simulink model "survillence"  (Simulink 7.9)
settings: Solver=ode45  StartTime=0.0  StopTime=100.0  RelTol=1e-3
undefined symbols (not defined in the file): jet
libraries: visionsinks x2, visionanalysis x1, dspvision x1
settings Model: Creator=user  LastModifiedBy=user

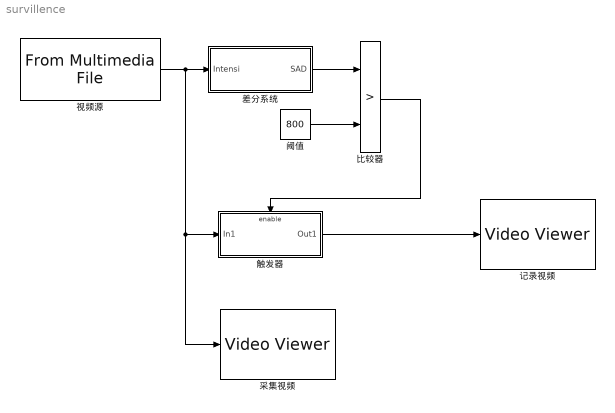
== system survillence ==
  差分系统 : Subsystem
  比较器 : RelationalOperator  Operator=>  OutDataTypeStr=boolean
  视频源 : dspvision/From Multimedia File  inputFilename=vipmen.avi  loop=on  numPlays=inf  outputStreams=Video only  videoDataType=double  audioDataType=int16  inheritSampleTime=on  userDefinedSampleTime=1/30  noAudioOutput=off  isIntensityVideo=off  fourcc=Intensity  colorVideoFormat=One multidimensional signal  outputEOF=off  dataOrg=Column-major  audioFrameSize=1024  computeAudioFrameSize=off  outSamplingMode=Sample based
  触发器 : Subsystem
  记录视频 : visionsinks/Video Viewer  inputType=Obsolete7b  imagePorts=One multidimensional signal  useColorMap=off  colormapValue=jet(256)  specRange=off  minInputVal=0  maxInputVal=255  FigPos=[601 774 410 300]  AxisZoom=on  trueSizedOnce=off  OpenAtMdlStart=on
  采集视频 : visionsinks/Video Viewer  inputType=Obsolete7b  imagePorts=One multidimensional signal  useColorMap=off  colormapValue=jet(256)  specRange=off  minInputVal=0  maxInputVal=255  FigPos=[78 1062 410 300]  AxisZoom=on  trueSizedOnce=off  OpenAtMdlStart=on
  阈值 : Constant  Value=800  VectorParams1D=off
  wires:
  视频源/1 -> 差分系统/1(Intensi), 触发器/1(In1), 采集视频/1
  阈值/1 -> 比较器/2
  差分系统/1(SAD) -> 比较器/1
  比较器/1 -> 触发器/Enable
  触发器/1(Out1) -> 记录视频/1

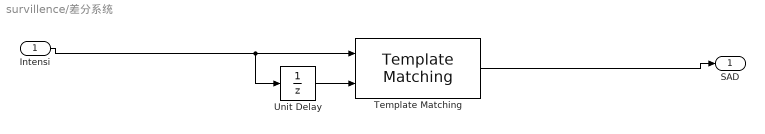
== system survillence/差分系统 ==
  Intensi : Inport
  Template Matching : visionanalysis/Template Matching  metric=Sum of absolute differences  output=Metric matrix  method=Exhaustive  nMetric=off  nSize=3  roi=off  roiValid=off  accumMode=Binary point scaling  accumWordLength=32  accumFracLength=0  prodOutputMode=Binary point scaling  prodOutputWordLength=32  prodOutputFracLength=0  roundingMode=Floor  overflowMode=off
  Unit Delay : UnitDelay  SampleTime=-1
  SAD : Outport
  wires:
  Template Matching/1 -> SAD/1
  Intensi/1 -> Template Matching/1, Unit Delay/1
  Unit Delay/1 -> Template Matching/2

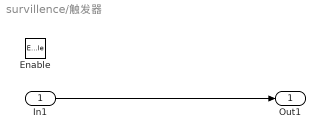
== system survillence/触发器 ==
  In1 : Inport
  Enable : EnablePort  PropagateVarSize=During execution
  Out1 : Outport
  wires:
  In1/1 -> Out1/1
